simulink model "flightGNCSim"  (R2021a)
settings: Solver=VariableStepAuto  StartTime=0.0  StopTime=10.0  RelTol=1e-3
values from neighbouring files (symbols this model uses):
  A = [Yv, Yp, -(u0 - Yr), c.g ... (first row only)    [dynamics_lab4_lat.m]    (also in dynamics_lab4_lon.m = [Xu, Xw, 0, -c.g;      Zu, Zw, u0, 0;      Mu + Mwd*Zu, Mw +; flightGNC.m = asind(wind * sind(alpha)/d); lat_dynamics.m; long_dynamics.m = [Xu, Xw, 0, -c.g;      Zu, Zw, u0, 0;      Mu + Mwd*Zu, Mw +)
  B = [Ydr, 0 ... (first row only)    [dynamics_lab4_lat.m]    (also in dynamics_lab4_lon.m = [Xde, XdT;      Zde, ZdT;      Mde + Mwd*Zde, MdT + Mwd*ZdT;; lat_dynamics.m; long_dynamics.m = [Xde, XdT;      Zde, ZdT;      Mde + Mwd*Zde, MdT + Mwd*ZdT;; ssModel.m = 1)
  D = pracNF .* sind(AoA) + pracAF .* cosd(AoA)    [analysisA.m]
  K = 0.5    [ssModel.m]
undefined symbols (not defined in the file or in its folder): C
settings Model: Creator=chilla  LastModifiedBy=chilla

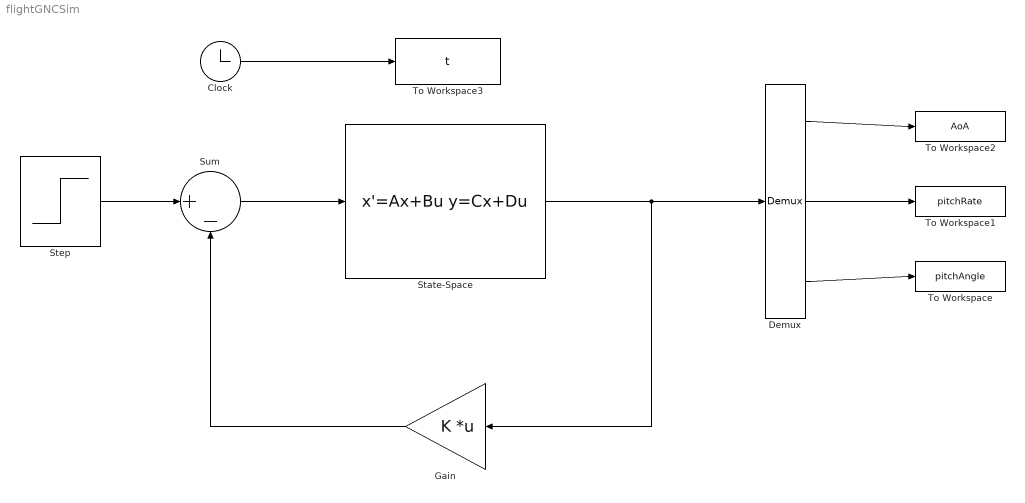
== system flightGNCSim ==
  Clock : Clock
  Demux : Demux  Outputs=3
  Gain : Gain  Gain=K  Multiplication=Matrix(K*u)
  State-Space : StateSpace  A=A  B=B  C=C  D=D  InitialCondition=0  ContinuousStateAttributes={'AoA', 'Pitch_Rate', 'Pitch_Angle'}
  Step : Step  Before=1  SampleTime=0
  Sum : Sum  Inputs=|+-
  To Workspace : ToWorkspace  VariableName=pitchAngle  SampleTime=-1
  To Workspace1 : ToWorkspace  VariableName=pitchRate  SampleTime=-1
  To Workspace2 : ToWorkspace  VariableName=AoA  SampleTime=-1
  To Workspace3 : ToWorkspace  VariableName=t  SampleTime=-1
  wires:
  State-Space/1 -> Gain/1, Demux/1
  Demux/1 -> To Workspace2/1
  Demux/2 -> To Workspace1/1
  Demux/3 -> To Workspace/1
  Step/1 -> Sum/1
  Sum/1 -> State-Space/1
  Gain/1 -> Sum/2
  Clock/1 -> To Workspace3/1
